simulink model "second"  (R2023b)
settings: Solver=FixedStepAuto  StartTime=0.0  StopTime=5  FixedStep=0.001  RelTol=1e-3
values from neighbouring files (symbols this model uses):
  A = [-1 0 0 0 ... (first row only)    [untitled.m]    (also in untitled2.m)
undefined symbols (not defined in the file or in its folder): C, L, x0, x1
settings Model: Creator=evdokiiagalkina  LastModifiedBy=evdokiiagalkina

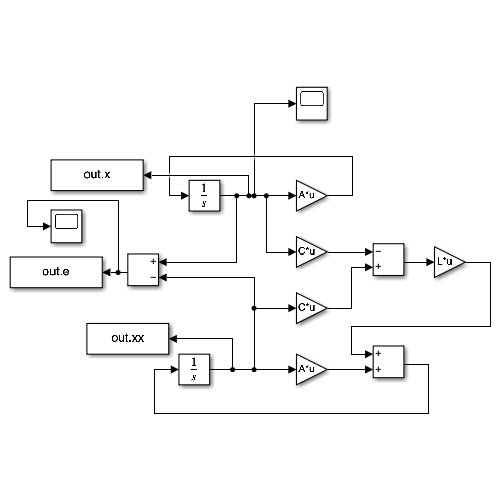
[thumbnail: Simulink's stored preview of the top-level diagram]
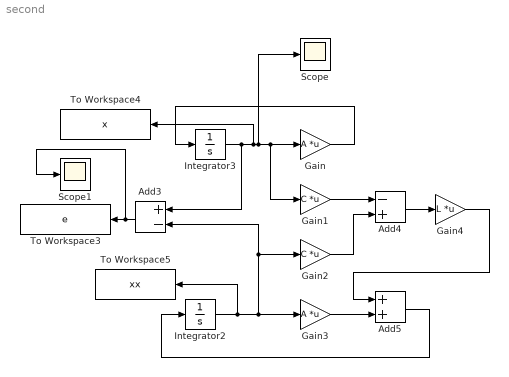
== system second ==
  Add3 : Sum  Inputs=+-
  Add4 : Sum  Inputs=-+
  Add5 : Sum
  Gain : Gain  Gain=A  Multiplication=Matrix(K*u)
  Gain1 : Gain  Gain=C  Multiplication=Matrix(K*u)
  Gain2 : Gain  Gain=C  Multiplication=Matrix(K*u)
  Gain3 : Gain  Gain=A  Multiplication=Matrix(K*u)
  Gain4 : Gain  Gain=L  Multiplication=Matrix(K*u)
  Integrator2 : Integrator  InitialCondition=x1
  Integrator3 : Integrator  InitialCondition=x0
  Scope : Scope
  Scope1 : Scope
  To Workspace3 : ToWorkspace  VariableName=e  SaveFormat=Timeseries  SampleTime=-1
  To Workspace4 : ToWorkspace  VariableName=x  SaveFormat=Timeseries  SampleTime=-1
  To Workspace5 : ToWorkspace  VariableName=xx  SaveFormat=Timeseries  SampleTime=-1
  wires:
  Integrator3/1 -> Add3/1, To Workspace4/1, Scope/1, Gain1/1, Gain/1
  Gain/1 -> Integrator3/1
  Gain1/1 -> Add4/1
  Gain2/1 -> Add4/2
  Integrator2/1 -> To Workspace5/1, Gain3/1, Add3/2, Gain2/1
  Gain3/1 -> Add5/2
  Add5/1 -> Integrator2/1
  Add3/1 -> Scope1/1, To Workspace3/1
  Add4/1 -> Gain4/1
  Gain4/1 -> Add5/1
